simulink model "Kalman_Tuning"  (R2019a)
settings: Solver=ode1  StartTime=0.0  StopTime=finalTime  FixedStep=sampleTime  RelTol=1e-3
undefined symbols (not defined in the file or in its folder): DiscIntNeverNeededParam, Kalman_OP, sampleTime
settings Model: Creator=Gaming  LastModifiedBy=Gaming

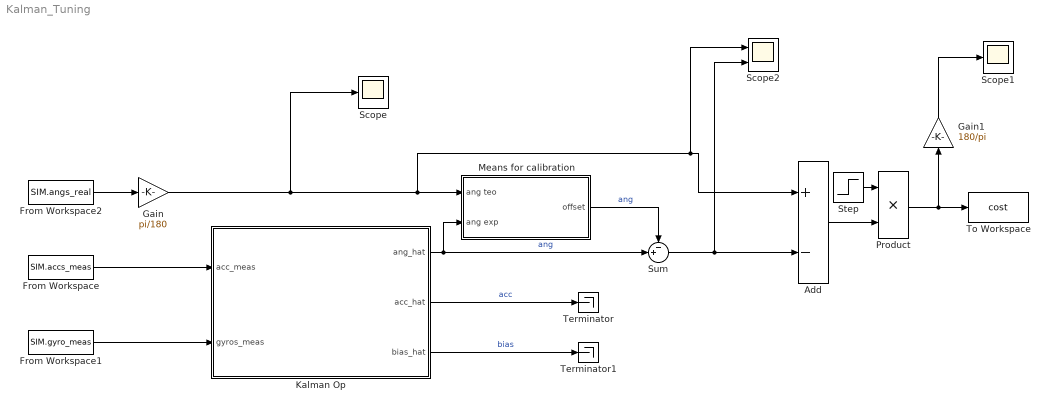
== system Kalman_Tuning ==
  Add : Sum  Inputs=+-
  From Workspace : FromWorkspace  VariableName=SIM.accs_meas  SampleTime=0
  From Workspace1 : FromWorkspace  VariableName=SIM.gyro_meas  SampleTime=0
  From Workspace2 : FromWorkspace  VariableName=SIM.angs_real  SampleTime=0
  Gain : Gain  Gain=pi/180
  Gain1 : Gain  Gain=180/pi
  Kalman Op : Subsystem
  Means for calibration : Subsystem
  Product : Product
  Scope : Scope
  Scope1 : Scope
  Scope2 : Scope  NumInputPorts=2
  Step : Step  Time=3.5  SampleTime=sampleTime
  Sum : Sum  Inputs=-+|
  Terminator : Terminator
  Terminator1 : Terminator
  To Workspace : ToWorkspace  VariableName=cost  SampleTime=-1
  wires:
  From Workspace/1 -> Kalman Op/1(acc_meas)
  From Workspace1/1 -> Kalman Op/2(gyros_meas)
  Kalman Op/3(bias_hat) -> Terminator1/1  "bias"
  Kalman Op/2(acc_hat) -> Terminator/1  "acc"
  Product/1 -> To Workspace/1, Gain1/1
  Kalman Op/1(ang_hat) -> Sum/2, Means for calibration/2(ang exp)  "ang"
  Add/1 -> Product/2
  Step/1 -> Product/1
  From Workspace2/1 -> Gain/1
  Gain/1 -> Scope2/1, Add/1, Means for calibration/1(ang teo), Scope/1
  Sum/1 -> Scope2/2, Add/2
  Means for calibration/1(offset) -> Sum/1  "ang"
  Gain1/1 -> Scope1/1

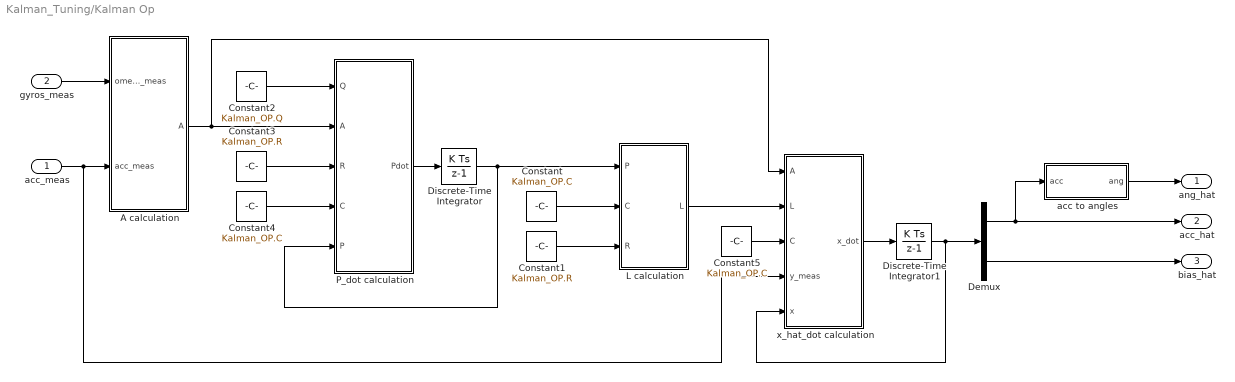
== system Kalman_Tuning/Kalman Op ==
  acc_meas : Inport
  gyros_meas : Inport  Port=2
  A calculation : MATLAB Function  TreatAsAtomicUnit=on
  Constant : Constant  Value=Kalman_OP.C
  Constant1 : Constant  Value=Kalman_OP.R
  Constant2 : Constant  Value=Kalman_OP.Q
  Constant3 : Constant  Value=Kalman_OP.R
  Constant4 : Constant  Value=Kalman_OP.C
  Constant5 : Constant  Value=Kalman_OP.C
  Demux : Demux  Outputs=2
  Discrete-Time Integrator : DiscreteIntegrator  InitialCondition=Kalman_OP.Q*10  SampleTime=-1  ICPrevOutput=DiscIntNeverNeededParam  ICPrevScaledInput=DiscIntNeverNeededParam
  Discrete-Time Integrator1 : DiscreteIntegrator  InitialCondition=zeros(6,1)  SampleTime=-1  ICPrevOutput=DiscIntNeverNeededParam  ICPrevScaledInput=DiscIntNeverNeededParam
  L calculation : MATLAB Function  TreatAsAtomicUnit=on
  P_dot calculation : MATLAB Function  TreatAsAtomicUnit=on
  acc to angles : MATLAB Function  TreatAsAtomicUnit=on
  x_hat_dot calculation : MATLAB Function  TreatAsAtomicUnit=on
  ang_hat : Outport
  acc_hat : Outport  Port=2
  bias_hat : Outport  Port=3
  wires:
  acc to angles/1(ang) -> ang_hat/1
  x_hat_dot calculation/1(x_dot) -> Discrete-Time Integrator1/1
  Discrete-Time Integrator1/1 -> Demux/1, x_hat_dot calculation/5(x)
  L calculation/1(L) -> x_hat_dot calculation/2(L)
  P_dot calculation/1(Pdot) -> Discrete-Time Integrator/1
  Discrete-Time Integrator/1 -> P_dot calculation/5(P), L calculation/1(P)
  Constant/1 -> L calculation/2(C)
  Constant1/1 -> L calculation/3(R)
  Constant3/1 -> P_dot calculation/3(R)
  Constant2/1 -> P_dot calculation/1(Q)
  Demux/1 -> acc to angles/1(acc), acc_hat/1
  Demux/2 -> bias_hat/1
  acc_meas/1 -> x_hat_dot calculation/4(y_meas), A calculation/2(acc_meas)
  gyros_meas/1 -> A calculation/1(omega_meas)
  A calculation/1(A) -> x_hat_dot calculation/1(A), P_dot calculation/2(A)
  Constant4/1 -> P_dot calculation/4(C)
  Constant5/1 -> x_hat_dot calculation/3(C)

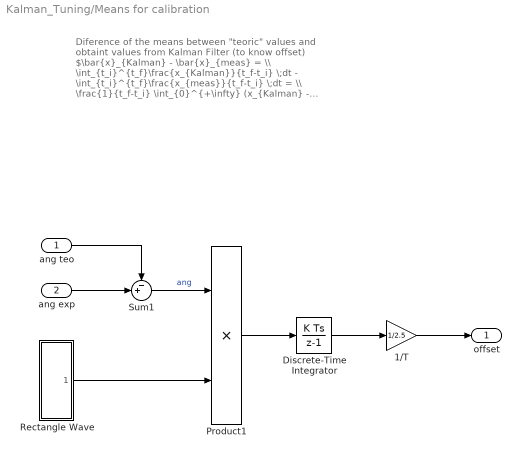
== system Kalman_Tuning/Means for calibration ==
  note: Diference of the means between "teoric" values and obtaint values from Kalman Filter (to know offset)
      |
      | $\bar{x}_{Kalman} - \bar{x}_{meas} = \\ \int_{t_i}^{t_f}\frac{x_{Kalman}}{t_f-t_i} \;dt - \int_{t_i}^{t_f}\frac{x_{meas}}{t_f-t_i} \;dt = \\ \frac{1}{t_f-t_i} \int_{0}^{+\infty} (x_{Kalman} - x_{meas})*\Pi \;dt$
  ang teo : Inport
  ang exp : Inport  Port=2
  1/T : Gain  Gain=1/2.5
  Discrete-Time Integrator : DiscreteIntegrator  SampleTime=-1  ICPrevOutput=DiscIntNeverNeededParam  ICPrevScaledInput=DiscIntNeverNeededParam
  Product1 : Product
  Rectangle Wave : Subsystem
  Sum1 : Sum  Inputs=-+|
  offset : Outport  VectorParamsAs1DForOutWhenUnconnected=on
  wires:
  Discrete-Time Integrator/1 -> 1/T/1
  ang exp/1 -> Sum1/2
  ang teo/1 -> Sum1/1
  Sum1/1 -> Product1/1  "ang"
  Product1/1 -> Discrete-Time Integrator/1
  1/T/1 -> offset/1
  Rectangle Wave/1(Pulse) -> Product1/2

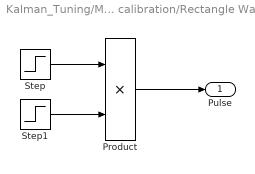
== system Kalman_Tuning/Means for calibration/Rectangle Wave ==
  Product : Product
  Step : Step  Time=0.5  SampleTime=0
  Step1 : Step  Time=3  Before=1  After=0  SampleTime=0
  Pulse : Outport
  wires:
  Step/1 -> Product/1
  Step1/1 -> Product/2
  Product/1 -> Pulse/1

== matlab function Kalman_Tuning/Kalman Op/A calculation ==
  data: omega_meas input; A output; acc_meas input
function A = fcn(omega_meas, acc_meas)

w = omega_meas;
a = acc_meas;

s_1 = [ 0   , -w(3) ,  w(2) ;...
        w(3),  0    , -w(1) ;...
       -w(2),  w(1) ,  0    ];
   
s_2 = [ 0   , -a(3) ,  a(2) ;...
        a(3),  0    , -a(1) ;...
       -a(2),  a(1) ,  0    ];
   
A = [-s_1, -s_2 ;...
     zeros(3,6) ];

== matlab function Kalman_Tuning/Kalman Op/P_dot calculation ==
  data: Q input; A input; Pdot output; R input; C input; P input
function Pdot = fcn(Q, A, R, C, P)

Pdot = A*P + P*transpose(A) + Q - P*transpose(C)*inv(R)*C*P;

== matlab function Kalman_Tuning/Kalman Op/acc to angles ==
  data: acc input; ang output
function ang = fcn(acc)

phi = -atan2(acc(2),-acc(3));

theta = atan2(acc(1),sqrt(acc(2)^2+acc(3)^2));

ang = [phi; theta];

== matlab function Kalman_Tuning/Kalman Op/L calculation ==
  data: P input; L output; C input; R input
function L = fcn(P, C, R)

L = P*transpose(C)*inv(R);

== matlab function Kalman_Tuning/Kalman Op/x_hat_dot calculation ==
  data: A input; x_dot output; L input; C input; y_meas input; x input
function x_dot = fcn(A,L,C,y_meas,x)

x_dot = A*x + L*(y_meas - C*x);
